simulink model "SoRo_Crt_SMM_20240410"  (R2023a)
settings: Solver=FixedStepAuto  StartTime=0.0  StopTime=50  FixedStep=0.01  RelTol=1e-3
PreLoadFcn:
  | load('traj_pos.mat')
undefined symbols (not defined in the file or in its folder): canChannel
libraries: simulink x18, canmsglib x14, canlib x11, dspfdesign x10, slpidlib x8, auroraNDILibrary x1
(part 1 of 2)
settings Model: Creator=86188  LastModifiedBy=86188
settings DebuggingCC: AlgebraicLoopMsg=none

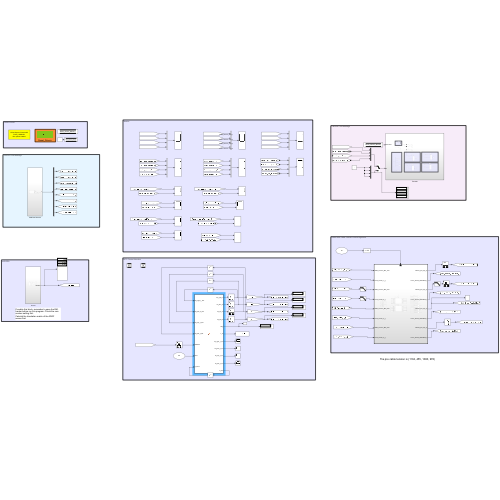
[thumbnail: Simulink's stored preview of the top-level diagram]
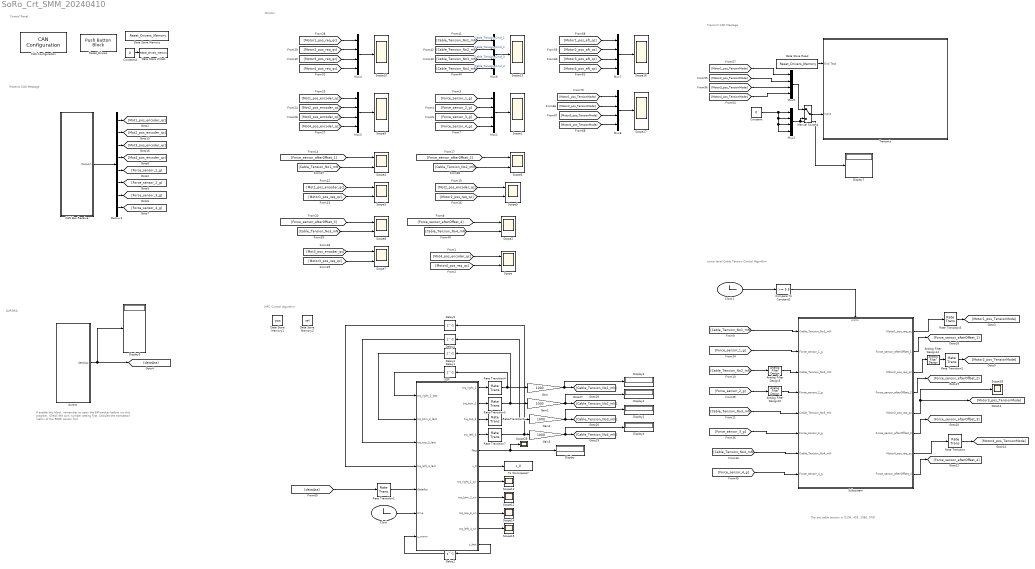
== system SoRo_Crt_SMM_20240410 ==
  note: The pre cable tension is (1104, 455, 1080, 978)
  note: AURORA
  note: If enable this block, remember to open the EM-tracker before run this program. Check the com number setting first.
      | Calculat the translation matrix of the 5DOF sensor first.
  note: Monitor
  note: Control Panel
  note: Lower level Cable Tension Control Algorithm
  note: Receive CAN Message
  note: Transmit CAN Message
  note: MPC Control Algorithm
  Analog Filter Design10 : dspfdesign/Analog Filter Design  method=Butterworth  filttype=Lowpass  N=3  Wlo=20  Whi=80  Rp=2  Rs=40
  Analog Filter Design14 : dspfdesign/Analog Filter Design  method=Butterworth  filttype=Lowpass  N=3  Wlo=20  Whi=80  Rp=2  Rs=40
  Analog Filter Design5 : dspfdesign/Analog Filter Design  method=Butterworth  filttype=Lowpass  N=3  Wlo=20  Whi=80  Rp=2  Rs=40
  Aurora : Subsystem
  CAN Bus Receive : Subsystem
  CAN Configuration : canlib/CAN Configuration  BlockHandle=2496.0005  Device=PEAK-System PCAN-USB (PCAN_USBBUS1)  DeviceMenu=PEAK-System PCAN-USB (PCAN_USBBUS1)  ObjConstructor=canChannel('PEAK-System', 'PCAN_USBBUS1')  BusSpeed=500000  EnableBitParameters=off  AckMode=Normal
  Clock : Clock
  Clock1 : Clock
  Compare To Constant2 : simulink/Logic and Bit Operations/Compare To Constant  relop=>=  const=5.5  OutDataTypeStr=boolean
  Constant : Constant  Value=0
  Constant4 : Constant  Value=0
  Data Store Memory : DataStoreMemory  DataStoreName=Reset_Drivers_Memory  ReadBeforeWriteMsg=warning  WriteAfterWriteMsg=warning  WriteAfterReadMsg=warning  ShowAdditionalParam=off
  Data Store Memory1 : DataStoreMemory  DataStoreName=pos  WriteAfterWriteMsg=warning  InitialValue=pos  ShowAdditionalParam=off  OutDataTypeStr=double
  Data Store Memory2 : DataStoreMemory  DataStoreName=vel  WriteAfterWriteMsg=warning  InitialValue=pos  ShowAdditionalParam=off  OutDataTypeStr=double
  Data Store Read : DataStoreRead  DataStoreName=Reset_Drivers_Memory  DataStoreElements=Reset_Drivers_Memory  IndexOptions=Index vector (dialog)  Indices=1  OutputSizes=1
  Data Store Write1 : DataStoreWrite  DataStoreName=Reset_Drivers_Memory  DataStoreElements=Reset_Drivers_Memory  IndexOptions=Index vector (dialog)  Indices=1  OutputSizes=1
  Delay1 : Delay  DelayLength=1  InitialCondition=0.001
  Delay2 : Delay  DelayLength=1  InitialCondition=|
      | [0.00100000000000000
      | 0.00100000000000000
      | 0.500800000000000
      | 0.00100000000000000
      | 0.00100000000000000
      | 0.00100000000000000
      | 0.500800000000000
      | 0.00100000000000000
      | 0.00100000000000000
      | 0.00100000000000000
      | 0.500800000000000
      | 0.00100000000000000
      | 0.00100000000000000
      | 0.00100000000000000
      | 0.500800000000000
      | 0.00100000000000000
      | 0.00100000000000000
      | 0.00100000000000000
      | 0.500800000000000
      | 0.00100000000000000
      | 0.00100000000000000
      | 0.00100000000000000
      | 0.500800000000000
      | 0.00100000000000000
      | 0.00100000000000000
      | 0.00100000000000000
      | 0.500800000000000
      | 0.00100000000000000
      | 0.00100000000000000
      | 0.00100000000000000
      | 0.500800000000000
      | 0.00100000000000000
      | 0.00100000000000000
      | 0.00100000000000000
      | 0.500800000000000
      | 0.00100000000000000
      | 0.00100000000000000
      | 0.00100000000000000
      | 0.500800000000000
      | 0.00100000000000000
      | -0.136300000000000
      | -0.384000000000000
      | -0.0157000000000000
      | -0.136300000000000
      | -0.384000000000000
      | -0.0157000000000000
      | -0.136300000000000
      | -0.384000000000000
      | -0.0157000000000000
      | -0.136300000000000
      | -0.384000000000000
      | -0.0157000000000000
      | -0.136300000000000
      | -0.384000000000000
      | -0.0157000000000000
      | -0.136300000000000
      | -0.384000000000000
      | -0.0157000000000000
      | -0.136300000000000
      | -0.384000000000000
      | -0.0157000000000000
      | -0.136300000000000
      | -0.384000000000000
      | -0.0157000000000000
      | -0.136300000000000
      | -0.384000000000000
      | -0.0157000000000000
      | -0.136300000000000
      | -0.384000000000000
      | -0.0157000000000000
      | 0
      | 0
      | 0
      | 0
      | 0
      | 0
      | 0
      | 0
      | 0
      | 0]
  Delay3 : Delay  DelayLength=1  InitialCondition=0.001
  Delay4 : Delay  DelayLength=1  InitialCondition=0.5008
  Delay5 : Delay  DelayLength=1  InitialCondition=0.001
  Demux1 : Demux  Outputs=8
  Display{,1..5,7} (7 alike) : Display
  Gain{,1..3} (4 alike) : Gain  Gain=1000
  Manual Switch4 : ManualSwitch
  Mux{1..8} (8 alike) : Mux
  Rate Transition{,2..3,5,7} (5 alike) : RateTransition  OutPortSampleTime=0.01
  Rate Transition1 : RateTransition  OutPortSampleTime=0.05
  Rate Transition4 : RateTransition  InitialCondition=0.001  OutPortSampleTime=0.01
  Rate Transition6 : RateTransition  InitialCondition=0.5008  OutPortSampleTime=0.01
  Reset_Drivers : PushButtonBlock  OffValue=0.000000
  SQP : MATLAB Function  TreatAsAtomicUnit=on
  Scope{,2..8} (8 alike) : Scope  NumInputPorts=2
  Scope{1,9..18,28} (12 alike) : Scope
  Subsystem : Subsystem
  To Workspace7 : ToWorkspace  VariableName=x_0  SaveFormat=Timeseries  SampleTime=-1
  Transmit : Subsystem
  wires:
  CAN Bus Receive/1(Outport) -> Demux1/1
  Constant4/1 -> Data Store Write1/1
  Data Store Read/1 -> Transmit/1(End Test)
  Demux1/1 -> [Mot1_pos_encoder_qc]
  Demux1/2 -> [Mot2_pos_encoder_qc]
  Demux1/3 -> [Mot3_pos_encoder_qc]
  Demux1/4 -> [Mot4_pos_encoder_qc]
  Demux1/5 -> [Force_sensor_1_g]
  Demux1/6 -> [Force_sensor_2_g]
  Demux1/7 -> [Force_sensor_3_g]
  Demux1/8 -> [Force_sensor_4_g]
  Mux2/1 -> Manual Switch4/2, Display7/1
  [Mot4_pos_encoder_qc] -> Scope/1
  [Motor4_pos_req_qc] -> Scope/2
  Constant/1 -> Mux2/3, Mux2/4, Mux2/2, Mux2/1
  [Motor1_pos_req_qc] -> Scope3/2
  [Cable_Tension_No1_mN] -> Scope4/2
  [Force_sensor_afterOffset_1] -> Scope4/1
  [Mot1_pos_encoder_qc] -> Scope3/1
  [Mot2_pos_encoder_qc] -> Scope5/1
  [Motor2_pos_req_qc] -> Scope5/2
  [Mot3_pos_encoder_qc] -> Scope7/1
  [Motor3_pos_req_qc] -> Scope7/2
  [Force_sensor_1_g] -> Mux1/1
  [Force_sensor_2_g] -> Mux1/2
  [Force_sensor_3_g] -> Mux1/3
  [Force_sensor_4_g] -> Mux1/4
  Mux1/1 -> Scope1/1
  Mux3/1 -> Scope9/1
  [Mot4_pos_encoder_qc] -> Mux3/4
  [Mot3_pos_encoder_qc] -> Mux3/3
  [Mot2_pos_encoder_qc] -> Mux3/2
  [Mot1_pos_encoder_qc] -> Mux3/1
  Mux4/1 -> Scope10/1
  [Motor4_pos_req_qc] -> Mux4/4
  [Motor3_pos_req_qc] -> Mux4/3
  [Motor2_pos_req_qc] -> Mux4/2
  [Motor1_pos_req_qc] -> Mux4/1
  Manual Switch4/1 -> Transmit/2(Input)
  Mux5/1 -> Manual Switch4/1
  [Motor2_pos_TensionMode] -> Mux5/2
  [Motor3_pos_TensionMode] -> Mux5/3
  Aurora/1(dataAss) -> Display5/1, [dataAss]
  [Force_sensor_afterOffset_2] -> Scope6/1
  [Cable_Tension_No2_mN] -> Scope6/2
  [Force_sensor_afterOffset_3] -> Scope8/1
  [Cable_Tension_No3_mN] -> Scope8/2
  [Cable_Tension_No4_mN] -> Scope2/2
  [Force_sensor_afterOffset_4] -> Scope2/1
  [Cable_Tension_No1_mN] -> Mux6/1  "Cable_Tension_Cmd_1"
  [Cable_Tension_No2_mN] -> Mux6/2  "Cable_Tension_Cmd_2"
  [Cable_Tension_No3_mN] -> Mux6/3  "Cable_Tension_Cmd_3"
  [Cable_Tension_No4_mN] -> Mux6/4  "Cable_Tension_Cmd_4"
  Mux6/1 -> Scope13/1
  Clock1/1 -> Compare To Constant2/1
  Compare To Constant2/1 -> Subsystem/Enable
  [Cable_Tension_No2_mN] -> Analog Filter Design5/1
  [Force_sensor_2_g] -> Analog Filter Design10/1
  Subsystem/3(Motor2_pos_req_qc) -> Analog Filter Design14/1
  Subsystem/2(Force_sensor_afterOffset_1) -> [Force_sensor_afterOffset_1]
  Subsystem/4(Force_sensor_afterOffset_2) -> [Force_sensor_afterOffset_2]
  Subsystem/6(Force_sensor_afterOffset_3) -> [Force_sensor_afterOffset_3]
  Subsystem/8(Force_sensor_afterOffset_4) -> [Force_sensor_afterOffset_4]
  [Motor1_pos_aft_qc] -> Mux7/1
  [Motor3_pos_aft_qc] -> Mux7/3
  [Motor2_pos_aft_qc] -> Mux7/2
  Mux7/1 -> Scope16/1
  [Motor4_pos_aft_qc] -> Mux7/4
  [Cable_Tension_No1_mN] -> Subsystem/1(Cable_Tension_No1_mN)
  Analog Filter Design5/1 -> Subsystem/3(Cable_Tension_No2_mN)
  [Cable_Tension_No3_mN] -> Subsystem/5(Cable_Tension_No3_mN)
  [Cable_Tension_No4_mN] -> Subsystem/7(Cable_Tension_No4_mN)
  [Force_sensor_1_g] -> Subsystem/2(Force_sensor_1_g)
  Analog Filter Design10/1 -> Subsystem/4(Force_sensor_2_g)
  [Force_sensor_3_g] -> Subsystem/6(Force_sensor_3_g)
  [Force_sensor_4_g] -> Subsystem/8(Force_sensor_4_g)
  [Motor4_pos_TensionMode] -> Mux8/4
  Mux8/1 -> Scope17/1
  [Motor2_pos_TensionMode] -> Mux8/2
  [Motor3_pos_TensionMode] -> Mux8/3
  [Motor1_pos_TensionMode] -> Mux8/1
  Subsystem/1(Motor1_pos_req_qc) -> Rate Transition3/1
  Analog Filter Design14/1 -> Rate Transition2/1
  Subsystem/7(Motor4_pos_req_qc) -> Rate Transition/1
  Rate Transition/1 -> [Motor4_pos_TensionMode]
  Subsystem/5(Motor3_pos_req_qc) -> Scope18/1, [Motor3_pos_TensionMode]
  Rate Transition2/1 -> [Motor2_pos_TensionMode]
  Rate Transition3/1 -> [Motor1_pos_TensionMode]
  [Motor1_pos_TensionMode] -> Mux5/1
  [Motor4_pos_TensionMode] -> Mux5/4
  SQP/1(trq_right_1) -> Rate Transition4/1
  SQP/2(trq_btm_2) -> Rate Transition5/1
  SQP/3(trq_top_3) -> Rate Transition6/1
  SQP/11(z_last) -> Delay2/1
  Clock/1 -> SQP/6(time)
  Delay2/1 -> SQP/7(z_warm)
  SQP/5(flag) -> Display/1, Scope28/1
  SQP/4(trq_left_4) -> Rate Transition7/1
  Rate Transition1/1 -> SQP/5(dataAss)
  Rate Transition4/1 -> Delay1/1, Gain/1
  Rate Transition5/1 -> Delay3/1, Gain1/1
  Rate Transition6/1 -> Delay4/1, Gain2/1
  Rate Transition7/1 -> Delay5/1, Gain3/1
  Gain/1 -> Display3/1, [Cable_Tension_No1_mN]
  Gain1/1 -> [Cable_Tension_No2_mN], Display2/1
  Gain3/1 -> [Cable_Tension_No4_mN], Display4/1
  [dataAss] -> Rate Transition1/1
  SQP/6(x_0) -> To Workspace7/1
  Gain2/1 -> Display1/1, [Cable_Tension_No3_mN]
  Delay1/1 -> SQP/1(trq_right_1_last)
  Delay3/1 -> SQP/2(trq_btm_2_last)
  Delay4/1 -> SQP/3(trq_top_3_last)
  Delay5/1 -> SQP/4(trq_left_4_last)
  SQP/7(trq_right_1_ori) -> Scope11/1
  SQP/8(trq_btm_2_ori) -> Scope12/1
  SQP/9(trq_top_3_ori) -> Scope14/1
  SQP/10(trq_left_4_ori) -> Scope15/1

== system SoRo_Crt_SMM_20240410/Aurora ==
  Aurora NDI Communication : auroraNDILibrary/Aurora NDI Communication  SampleFrequency=20  comNumber=5
  Clock : Clock
  Constant3 : Constant
  Display{1..4} (4 alike) : Display
  Goto5 : Goto  Commented=on  GotoTag=em_tracker_pos  TagVisibility=global
  Subsystem4 : Subsystem
      mask Display: disp('angle of two sensors');
  Subsystem5 : Subsystem  Commented=on
      mask Display: disp('tool1 in tool2');
  Terminator1 : Terminator
  Terminator4 : Terminator
  To Workspace : ToWorkspace  VariableName=DOF5  SaveFormat=Timeseries  SampleTime=-1
  To Workspace1 : ToWorkspace  VariableName=DOF6  SaveFormat=Timeseries  SampleTime=-1
  To Workspace7 : ToWorkspace  VariableName=dataAss  SaveFormat=Timeseries  SampleTime=-1
  t1 : Selector  Commented=on  NumberOfDimensions=2  InputPortWidth=11  IndexOptions=Index vector (dialog),Index vector (dialog)  Indices=[1: 3],4  OutputSizes=1,1
  dataAss : Outport
  wires:
  Aurora NDI Communication/3 -> Terminator1/1
  Aurora NDI Communication/2 -> Display3/1, Subsystem4/2(6DOF), To Workspace1/1
  Constant3/1 -> Aurora NDI Communication/Enable
  Aurora NDI Communication/1 -> Subsystem4/1(5DOF), Display4/1, To Workspace/1
  Aurora NDI Communication/5 -> Display1/1
  Clock/1 -> Aurora NDI Communication/1
  Aurora NDI Communication/4 -> Terminator4/1
  Subsystem5/1(Out1) -> t1/1
  t1/1 -> Goto5/1
  Subsystem4/1(dataAss) -> Display2/1, dataAss/1, To Workspace7/1

== system SoRo_Crt_SMM_20240410/CAN Bus Receive ==
  CAN Receive : canlib/CAN Receive  BlockHandle=2380.0005  Device=PEAK-System PCAN-USB (PCAN_USBBUS1)  DeviceMenu=PEAK-System PCAN-USB (PCAN_USBBUS1)  ObjConstructor=canChannel('PEAK-System', 'PCAN_USBBUS1')  EnableStandardIDsFilter=off  StdIDsCombo=Allow all  StandardIDs=0  EnableExtendedIDsFilter=off  ExtIDsCombo=Allow all  ExtendedIDs=0  SampleTime=0.01  MsgsPerTimestep=all  InternalFilterUpdateStatus=on  BusOutput=on
  Rate Transition : RateTransition  OutPortSampleTime=0.01
  Subsystem : Subsystem
  Outport : Outport
  wires:
  CAN Receive/2 -> Subsystem/1(In2)
  CAN Receive/1 -> Subsystem/Trigger
  Subsystem/1(Outport) -> Rate Transition/1
  Rate Transition/1 -> Outport/1

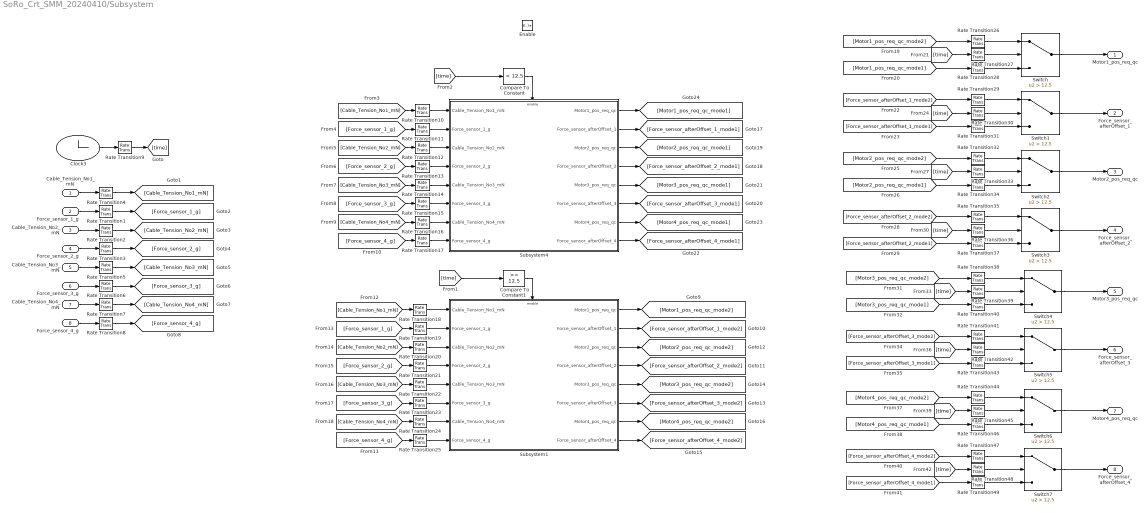
== system SoRo_Crt_SMM_20240410/Subsystem ==
  Cable_Tension_No1_mN : Inport
  Force_sensor_1_g : Inport  Port=2
  Cable_Tension_No2_mN : Inport  Port=3
  Force_sensor_2_g : Inport  Port=4
  Cable_Tension_No3_mN : Inport  Port=5
  Force_sensor_3_g : Inport  Port=6
  Cable_Tension_No4_mN : Inport  Port=7
  Force_sensor_4_g : Inport  Port=8
  Enable : EnablePort
  Clock3 : Clock
  Compare To Constant : simulink/Logic and Bit Operations/Compare To Constant  relop=<  const=12.5  OutDataTypeStr=boolean
  Compare To Constant1 : simulink/Logic and Bit Operations/Compare To Constant  relop=>=  const=12.5  OutDataTypeStr=boolean
  Rate Transition{1..49} (49 alike) : RateTransition  OutPortSampleTime=0.01
  Subsystem1 : Subsystem
  Subsystem4 : Subsystem
  Switch{,1..7} (8 alike) : Switch  Criteria=u2 > Threshold  Threshold=12.5  SaturateOnIntegerOverflow=off  InputSameDT=off
  Motor1_pos_req_qc : Outport
  Force_sensor_afterOffset_1 : Outport  Port=2
  Motor2_pos_req_qc : Outport  Port=3
  Force_sensor_afterOffset_2 : Outport  Port=4
  Motor3_pos_req_qc : Outport  Port=5
  Force_sensor_afterOffset_3 : Outport  Port=6
  Motor4_pos_req_qc : Outport  Port=7
  Force_sensor_afterOffset_4 : Outport  Port=8
  wires:
  Clock3/1 -> Rate Transition9/1
  Compare To Constant/1 -> Subsystem4/Enable
  [time] -> Compare To Constant/1
  Compare To Constant1/1 -> Subsystem1/Enable
  [time] -> Compare To Constant1/1
  [Cable_Tension_No1_mN] -> Rate Transition10/1
  [Force_sensor_1_g] -> Rate Transition11/1
  Cable_Tension_No1_mN/1 -> Rate Transition4/1
  Force_sensor_1_g/1 -> Rate Transition1/1
  Cable_Tension_No2_mN/1 -> Rate Transition2/1
  [Cable_Tension_No2_mN] -> Rate Transition12/1
  [Force_sensor_2_g] -> Rate Transition13/1
  Cable_Tension_No3_mN/1 -> Rate Transition5/1
  Force_sensor_3_g/1 -> Rate Transition6/1
  Cable_Tension_No4_mN/1 -> Rate Transition7/1
  Force_sensor_4_g/1 -> Rate Transition8/1
  Force_sensor_2_g/1 -> Rate Transition3/1
  [Cable_Tension_No3_mN] -> Rate Transition14/1
  [Force_sensor_3_g] -> Rate Transition15/1
  [Cable_Tension_No4_mN] -> Rate Transition16/1
  [Force_sensor_4_g] -> Rate Transition17/1
  [Cable_Tension_No2_mN] -> Rate Transition20/1
  [Force_sensor_2_g] -> Rate Transition21/1
  [Cable_Tension_No3_mN] -> Rate Transition22/1
  [Force_sensor_3_g] -> Rate Transition23/1
  [Cable_Tension_No4_mN] -> Rate Transition24/1
  [Force_sensor_4_g] -> Rate Transition25/1
  [Cable_Tension_No1_mN] -> Rate Transition18/1
  [Force_sensor_1_g] -> Rate Transition19/1
  Switch/1 -> Motor1_pos_req_qc/1
  [Motor1_pos_req_qc_mode2] -> Rate Transition26/1
  [Motor1_pos_req_qc_mode1] -> Rate Transition28/1
  [time] -> Rate Transition27/1
  [Force_sensor_afterOffset_1_mode1] -> Rate Transition31/1
  Switch1/1 -> Force_sensor_afterOffset_1/1
  [time] -> Rate Transition30/1
  [Force_sensor_afterOffset_1_mode2] -> Rate Transition29/1
  [time] -> Rate Transition33/1
  [Motor2_pos_req_qc_mode1] -> Rate Transition34/1
  [Motor2_pos_req_qc_mode2] -> Rate Transition32/1
  Switch2/1 -> Motor2_pos_req_qc/1
  [Force_sensor_afterOffset_2_mode2] -> Rate Transition35/1
  [time] -> Rate Transition36/1
  [Force_sensor_afterOffset_2_mode1] -> Rate Transition37/1
  Switch3/1 -> Force_sensor_afterOffset_2/1
  Switch4/1 -> Motor3_pos_req_qc/1
  [Motor3_pos_req_qc_mode1] -> Rate Transition40/1
  [Force_sensor_afterOffset_3_mode2] -> Rate Transition41/1
  [Motor3_pos_req_qc_mode2] -> Rate Transition38/1
  [time] -> Rate Transition39/1
  [time] -> Rate Transition42/1
  Switch5/1 -> Force_sensor_afterOffset_3/1
  [Force_sensor_afterOffset_3_mode1] -> Rate Transition43/1
  [Motor4_pos_req_qc_mode2] -> Rate Transition44/1
  [time] -> Rate Transition48/1
  [time] -> Rate Transition45/1
  [Force_sensor_afterOffset_4_mode1] -> Rate Transition49/1
  [Force_sensor_afterOffset_4_mode2] -> Rate Transition47/1
  [Motor4_pos_req_qc_mode1] -> Rate Transition46/1
  Switch7/1 -> Force_sensor_afterOffset_4/1
  Switch6/1 -> Motor4_pos_req_qc/1
  Subsystem1/1(Motor1_pos_req_qc) -> [Motor1_pos_req_qc_mode2]
  Subsystem1/2(Force_sensor_afterOffset_1) -> [Force_sensor_afterOffset_1_mode2]
  Subsystem1/3(Motor2_pos_req_qc) -> [Motor2_pos_req_qc_mode2]
  Subsystem1/4(Force_sensor_afterOffset_2) -> [Force_sensor_afterOffset_2_mode2]
  Subsystem1/5(Motor3_pos_req_qc) -> [Motor3_pos_req_qc_mode2]
  Subsystem1/6(Force_sensor_afterOffset_3) -> [Force_sensor_afterOffset_3_mode2]
  Subsystem1/7(Motor4_pos_req_qc) -> [Motor4_pos_req_qc_mode2]
  Subsystem1/8(Force_sensor_afterOffset_4) -> [Force_sensor_afterOffset_4_mode2]
  Subsystem4/1(Motor1_pos_req_qc) -> [Motor1_pos_req_qc_mode1]
  Subsystem4/2(Force_sensor_afterOffset_1) -> [Force_sensor_afterOffset_1_mode1]
  Subsystem4/3(Motor2_pos_req_qc) -> [Motor2_pos_req_qc_mode1]
  Subsystem4/4(Force_sensor_afterOffset_2) -> [Force_sensor_afterOffset_2_mode1]
  Subsystem4/5(Motor3_pos_req_qc) -> [Motor3_pos_req_qc_mode1]
  Subsystem4/6(Force_sensor_afterOffset_3) -> [Force_sensor_afterOffset_3_mode1]
  Subsystem4/7(Motor4_pos_req_qc) -> [Motor4_pos_req_qc_mode1]
  Subsystem4/8(Force_sensor_afterOffset_4) -> [Force_sensor_afterOffset_4_mode1]
  Rate Transition4/1 -> [Cable_Tension_No1_mN]
  Rate Transition1/1 -> [Force_sensor_1_g]
  Rate Transition2/1 -> [Cable_Tension_No2_mN]
  Rate Transition3/1 -> [Force_sensor_2_g]
  Rate Transition5/1 -> [Cable_Tension_No3_mN]
  Rate Transition6/1 -> [Force_sensor_3_g]
  Rate Transition7/1 -> [Cable_Tension_No4_mN]
  Rate Transition8/1 -> [Force_sensor_4_g]
  Rate Transition9/1 -> [time]
  Rate Transition10/1 -> Subsystem4/1(Cable_Tension_No1_mN)
  Rate Transition11/1 -> Subsystem4/2(Force_sensor_1_g)
  Rate Transition12/1 -> Subsystem4/3(Cable_Tension_No2_mN)
  Rate Transition13/1 -> Subsystem4/4(Force_sensor_2_g)
  Rate Transition14/1 -> Subsystem4/5(Cable_Tension_No3_mN)
  Rate Transition15/1 -> Subsystem4/6(Force_sensor_3_g)
  Rate Transition16/1 -> Subsystem4/7(Cable_Tension_No4_mN)
  Rate Transition17/1 -> Subsystem4/8(Force_sensor_4_g)
  Rate Transition18/1 -> Subsystem1/1(Cable_Tension_No1_mN)
  Rate Transition19/1 -> Subsystem1/2(Force_sensor_1_g)
  Rate Transition20/1 -> Subsystem1/3(Cable_Tension_No2_mN)
  Rate Transition21/1 -> Subsystem1/4(Force_sensor_2_g)
  Rate Transition22/1 -> Subsystem1/5(Cable_Tension_No3_mN)
  Rate Transition23/1 -> Subsystem1/6(Force_sensor_3_g)
  Rate Transition24/1 -> Subsystem1/7(Cable_Tension_No4_mN)
  Rate Transition25/1 -> Subsystem1/8(Force_sensor_4_g)
  Rate Transition26/1 -> Switch/1
  Rate Transition27/1 -> Switch/2
  Rate Transition28/1 -> Switch/3
  Rate Transition29/1 -> Switch1/1
  Rate Transition30/1 -> Switch1/2
  Rate Transition31/1 -> Switch1/3
  Rate Transition32/1 -> Switch2/1
  Rate Transition33/1 -> Switch2/2
  Rate Transition34/1 -> Switch2/3
  Rate Transition35/1 -> Switch3/1
  Rate Transition36/1 -> Switch3/2
  Rate Transition37/1 -> Switch3/3
  Rate Transition38/1 -> Switch4/1
  Rate Transition39/1 -> Switch4/2
  Rate Transition40/1 -> Switch4/3
  Rate Transition41/1 -> Switch5/1
  Rate Transition42/1 -> Switch5/2
  Rate Transition43/1 -> Switch5/3
  Rate Transition44/1 -> Switch6/1
  Rate Transition45/1 -> Switch6/2
  Rate Transition46/1 -> Switch6/3
  Rate Transition47/1 -> Switch7/1
  Rate Transition48/1 -> Switch7/2
  Rate Transition49/1 -> Switch7/3

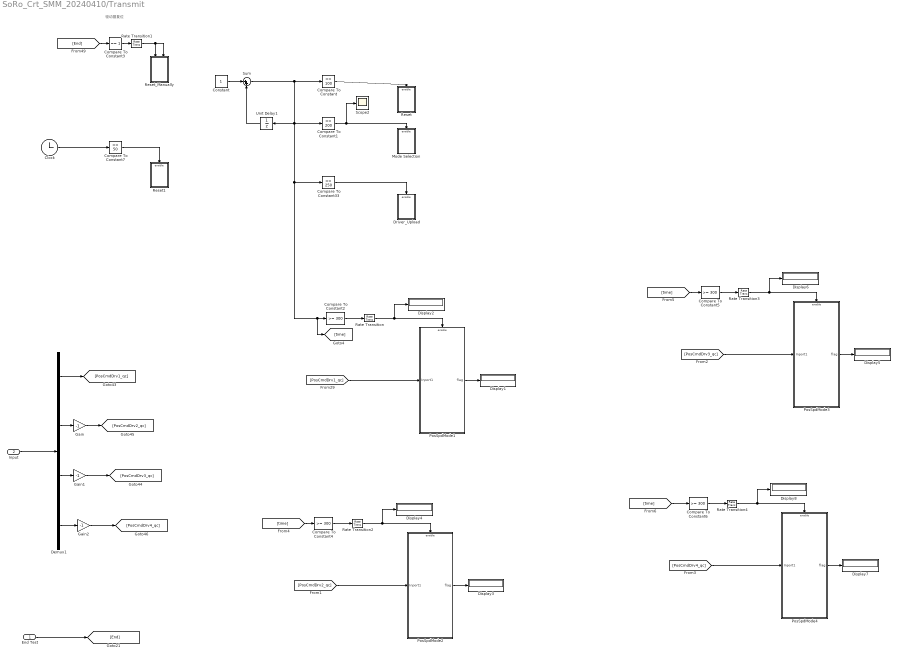
== system SoRo_Crt_SMM_20240410/Transmit ==
  note: 驱动器复位
  End Test : Inport
  Input : Inport  Port=2
  Clock : Clock
  Compare To Constant : simulink/Logic and Bit Operations/Compare To Constant  relop===  const=100  OutDataTypeStr=boolean
  Compare To Constant1 : simulink/Logic and Bit Operations/Compare To Constant  relop===  const=200  OutDataTypeStr=boolean
  Compare To Constant{2,4..6} (4 alike) : simulink/Logic and Bit Operations/Compare To Constant  relop=>=  const=300  OutDataTypeStr=boolean
  Compare To Constant3 : simulink/Logic and Bit Operations/Compare To Constant  relop===  const=1  OutDataTypeStr=boolean
  Compare To Constant33 : simulink/Logic and Bit Operations/Compare To Constant  relop===  const=250  OutDataTypeStr=boolean
  Compare To Constant7 : simulink/Logic and Bit Operations/Compare To Constant  relop===  const=50  OutDataTypeStr=boolean
  Constant : Constant
  Demux1 : Demux
  Display{1..8} (8 alike) : Display
  Driver_Upload : Subsystem
  Gain : Gain  Gain=-1
  Gain1 : Gain  Gain=-1
  Gain2 : Gain  Gain=-1
  Mode Selection : Subsystem  ScheduleAs=Aperiodic partition  PartitionName=TEMP_PRECOMP_PARTITION_NAME_MessageTriggeredSubsystem
  PosSpdMode1 : Subsystem
  PosSpdMode2 : Subsystem
  PosSpdMode3 : Subsystem
  PosSpdMode4 : Subsystem
  Rate Transition{,1..4} (5 alike) : RateTransition  OutPortSampleTime=1
  Reset : Subsystem
  Reset1 : Subsystem
  Reset_Manually : Subsystem
  Scope2 : Scope
  Sum : Sum  Inputs=|++  InputSameDT=on  SaturateOnIntegerOverflow=on  OutDataTypeStr=Inherit: Same as first input
  Unit Delay1 : UnitDelay  SampleTime=-1  HasFrameUpgradeWarning=on
  wires:
  Compare To Constant/1 -> Reset/Enable
  Compare To Constant1/1 -> Scope2/1, Mode Selection/Enable
  Compare To Constant2/1 -> Rate Transition/1
  Constant/1 -> Sum/1
  Unit Delay1/1 -> Sum/2
  Rate Transition/1 -> Display2/1, PosSpdMode1/Enable
  [End] -> Compare To Constant3/1
  [PosCmdDrv1_qc] -> PosSpdMode1/1(Inport1)
  Compare To Constant3/1 -> Rate Transition1/1
  Rate Transition1/1 -> Reset_Manually/Trigger, Reset_Manually/Enable
  Demux1/1 -> [PosCmdDrv1_qc]
  Demux1/3 -> Gain1/1
  Demux1/4 -> Gain2/1
  Input/1 -> Demux1/1
  Demux1/2 -> Gain/1
  End Test/1 -> [End]
  PosSpdMode1/1(flag) -> Display1/1
  PosSpdMode2/1(flag) -> Display3/1
  [PosCmdDrv2_qc] -> PosSpdMode2/1(Inport1)
  Rate Transition2/1 -> Display4/1, PosSpdMode2/Enable
  Compare To Constant4/1 -> Rate Transition2/1
  PosSpdMode3/1(flag) -> Display5/1
  [PosCmdDrv3_qc] -> PosSpdMode3/1(Inport1)
  Rate Transition3/1 -> Display6/1, PosSpdMode3/Enable
  Compare To Constant5/1 -> Rate Transition3/1
  PosSpdMode4/1(flag) -> Display7/1
  [PosCmdDrv4_qc] -> PosSpdMode4/1(Inport1)
  Rate Transition4/1 -> Display8/1, PosSpdMode4/Enable
  Compare To Constant6/1 -> Rate Transition4/1
  [time] -> Compare To Constant4/1
  [time] -> Compare To Constant5/1
  [time] -> Compare To Constant6/1
  Compare To Constant33/1 -> Driver_Upload/Enable
  Sum/1 -> [time], Compare To Constant2/1, Compare To Constant33/1, Compare To Constant1/1, Unit Delay1/1, Compare To Constant/1
  Gain/1 -> [PosCmdDrv2_qc]
  Gain1/1 -> [PosCmdDrv3_qc]
  Gain2/1 -> [PosCmdDrv4_qc]
  Compare To Constant7/1 -> Reset1/Enable
  Clock/1 -> Compare To Constant7/1

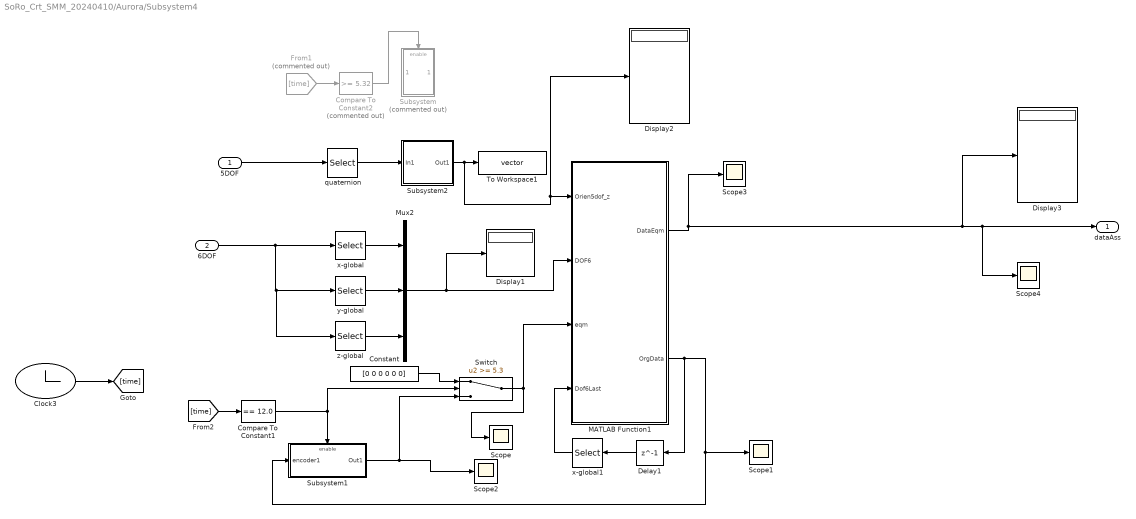
== system SoRo_Crt_SMM_20240410/Aurora/Subsystem4 ==
  5DOF : Inport
  6DOF : Inport  Port=2
  Clock3 : Clock
  Compare To Constant1 : simulink/Logic and Bit Operations/Compare To Constant  relop===  const=12.0  OutDataTypeStr=boolean
  Compare To Constant2 : simulink/Logic and Bit Operations/Compare To Constant  Commented=on  relop=>=  const=5.32  OutDataTypeStr=boolean
  Constant : Constant  Value=|
      | [0
      | 0
      | 0
      | 0
      | 0
      | 0]
  Delay1 : Delay  DelayLength=1  InitialCondition=[0; 0; 0; 0; 0; 0]
  Display1 : Display
  Display2 : Display
  Display3 : Display
  From1 : From  Commented=on  GotoTag=time
  MATLAB Function1 : MATLAB Function  TreatAsAtomicUnit=on
  Mux2 : Mux  Inputs=3
  Scope{,1..4} (5 alike) : Scope
  Subsystem : Subsystem  Commented=on
  Subsystem1 : Subsystem
  Subsystem2 : Subsystem
      mask Display: disp('z vector');
  Switch : Switch  Threshold=5.3  SaturateOnIntegerOverflow=off  InputSameDT=off
  To Workspace1 : ToWorkspace  VariableName=vector  SaveFormat=Timeseries  SampleTime=-1
  quaternion : Selector  InputPortWidth=7  IndexOptions=Index vector (dialog)  Indices=[1: 4]  OutputSizes=1
  x-global : Selector  InputPortWidth=7  IndexOptions=Index vector (dialog)  Indices=[5]  OutputSizes=1
  x-global1 : Selector  InputPortWidth=6  IndexOptions=Index vector (dialog)  Indices=[4:6]  OutputSizes=1
  y-global : Selector  InputPortWidth=7  IndexOptions=Index vector (dialog)  Indices=[6]  OutputSizes=1
  z-global : Selector  InputPortWidth=7  IndexOptions=Index vector (dialog)  Indices=[7]  OutputSizes=1
  dataAss : Outport
  wires:
  Subsystem2/1(Out1) -> Display2/1, MATLAB Function1/1(Orien5dof_z), To Workspace1/1
  quaternion/1 -> Subsystem2/1(In1)
  x-global/1 -> Mux2/1
  y-global/1 -> Mux2/2
  z-global/1 -> Mux2/3
  Switch/1 -> Scope/1, MATLAB Function1/3(eqm)
  6DOF/1 -> z-global/1, y-global/1, x-global/1
  5DOF/1 -> quaternion/1
  Compare To Constant1/1 -> Switch/2, Subsystem1/Enable
  [time] -> Compare To Constant1/1
  Mux2/1 -> Display1/1, MATLAB Function1/2(DOF6)
  MATLAB Function1/2(OrgData) -> Delay1/1, Subsystem1/1(encoder1), Scope1/1
  Subsystem1/1(Out1) -> Switch/3, Scope2/1
  Clock3/1 -> [time]
  Constant/1 -> Switch/1
  From1/1 -> Compare To Constant2/1
  Compare To Constant2/1 -> Subsystem/Enable
  MATLAB Function1/1(DataEqm) -> Display3/1, Scope4/1, dataAss/1, Scope3/1
  Delay1/1 -> x-global1/1
  x-global1/1 -> MATLAB Function1/4(Dof6Last)

== system SoRo_Crt_SMM_20240410/Aurora/Subsystem5 ==
  In1 : Inport
  In2 : Inport  Port=2
  Constant : Constant  Value=[0 0 0 1]  VectorParams1D=off
  Constant1 : Constant  Value=[0 0 0 1]  VectorParams1D=off
  Divide : Product  Inputs=*/  Multiplication=Matrix(*)
  Matrix Concatenate : Concatenate  Mode=Multidimensional array  ConcatenateDimension=2
  Matrix Concatenate1 : Concatenate  Mode=Multidimensional array
  Matrix Concatenate2 : Concatenate  Mode=Multidimensional array  ConcatenateDimension=2
  Matrix Concatenate3 : Concatenate  Mode=Multidimensional array
  Subsystem2 : Subsystem
      mask Display: disp('q2rot');
  Subsystem3 : Subsystem
      mask Display: disp('q2rot');
  q1 : Selector  InputPortWidth=11  IndexOptions=Index vector (dialog)  Indices=[4: 7]  OutputSizes=1
  q2 : Selector  InputPortWidth=11  IndexOptions=Index vector (dialog)  Indices=[4: 7]  OutputSizes=1
  t1 : Selector  InputPortWidth=11  IndexOptions=Index vector (dialog)  Indices=[8: 10]  OutputSizes=1
  t2 : Selector  InputPortWidth=11  IndexOptions=Index vector (dialog)  Indices=[8: 10]  OutputSizes=1
  Out1 : Outport
  wires:
  In2/1 -> t2/1, q2/1
  q2/1 -> Subsystem3/1(In1)
  q1/1 -> Subsystem2/1(In1)
  In1/1 -> t1/1, q1/1
  Subsystem2/1(Out1) -> Matrix Concatenate/1
  t1/1 -> Matrix Concatenate/2
  Matrix Concatenate/1 -> Matrix Concatenate1/1
  Constant/1 -> Matrix Concatenate1/2
  Constant1/1 -> Matrix Concatenate3/2
  Matrix Concatenate2/1 -> Matrix Concatenate3/1
  t2/1 -> Matrix Concatenate2/2
  Subsystem3/1(Out1) -> Matrix Concatenate2/1
  Matrix Concatenate1/1 -> Divide/1
  Matrix Concatenate3/1 -> Divide/2
  Divide/1 -> Out1/1

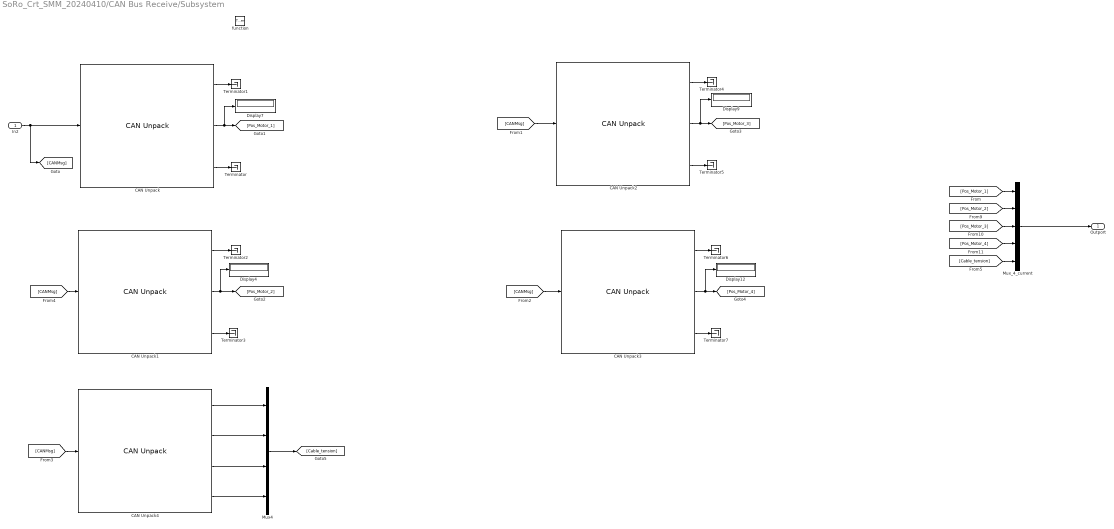
== system SoRo_Crt_SMM_20240410/CAN Bus Receive/Subsystem ==
  In2 : Inport
  function : TriggerPort  TriggerType=function-call  VariantControl=Variant
  CAN Unpack : canmsglib/CAN Unpack  CANdbFile=E:\Research\SRIL\9th\Mnp_Control_Sim\RoboModule0611.dbc  MsgList=Feedback_curvelpos_Dv1  MsgName=Feedback_curvelpos_Dv1  MsgIDType=Standard (11-bit identifier)  MsgIdentifier=27  MsgLength=8  SignalInfo={'real_current','8','16','BE','signed','Standard','0','1','0','-Inf','Inf';'real_position','56','32','BE','signed','Standard','0','1','0','-Inf','Inf';'real_velocity','24','16','BE','signed','Standard','0','1','0','-Inf','Inf'}  IDPort=off  TimestampPort=off  ErrorPort=off  RemotePort=off  LengthPort=off  StatusPort=off  ApplyMinMax=off
      settings: DataFormat=CANdb specified signals
  CAN Unpack1 : canmsglib/CAN Unpack  CANdbFile=E:\Research\SRIL\9th\Mnp_Control_Sim\RoboModule0611.dbc  MsgList=Feedback_curvelpos_Dv2  MsgName=Feedback_curvelpos_Dv2  MsgIDType=Standard (11-bit identifier)  MsgIdentifier=43  MsgLength=8  SignalInfo={'real_current','8','16','BE','signed','Standard','0','1','0','-Inf','Inf';'real_position','56','32','BE','signed','Standard','0','1','0','-Inf','Inf';'real_velocity','24','16','BE','signed','Standard','0','1','0','-Inf','Inf'}  IDPort=off  TimestampPort=off  ErrorPort=off  RemotePort=off  LengthPort=off  StatusPort=off  ApplyMinMax=off
      settings: DataFormat=CANdb specified signals
  CAN Unpack2 : canmsglib/CAN Unpack  CANdbFile=E:\Research\SRIL\9th\Mnp_Control_Sim\RoboModule0611.dbc  MsgList=Feedback_curvelpos_Dv3  MsgName=Feedback_curvelpos_Dv3  MsgIDType=Standard (11-bit identifier)  MsgIdentifier=59  MsgLength=8  SignalInfo={'real_current','8','16','BE','signed','Standard','0','1','0','-Inf','Inf';'real_position','56','32','BE','signed','Standard','0','1','0','-Inf','Inf';'real_velocity','24','16','BE','signed','Standard','0','1','0','-Inf','Inf'}  IDPort=off  TimestampPort=off  ErrorPort=off  RemotePort=off  LengthPort=off  StatusPort=off  ApplyMinMax=off
      settings: DataFormat=CANdb specified signals
  CAN Unpack3 : canmsglib/CAN Unpack  CANdbFile=E:\Research\SRIL\9th\Mnp_Control_Sim\RoboModule0611.dbc  MsgList=Feedback_curvelpos_Dr4  MsgName=Feedback_curvelpos_Dr4  MsgIDType=Standard (11-bit identifier)  MsgIdentifier=75  MsgLength=8  SignalInfo={'real_current','8','16','BE','signed','Standard','0','1','0','-Inf','Inf';'real_position','56','32','BE','signed','Standard','0','1','0','-Inf','Inf';'real_velocity','24','16','BE','signed','Standard','0','1','0','-Inf','Inf'}  IDPort=off  TimestampPort=off  ErrorPort=off  RemotePort=off  LengthPort=off  StatusPort=off  ApplyMinMax=off
      settings: DataFormat=CANdb specified signals
  CAN Unpack4 : canmsglib/CAN Unpack  CANdbFile=E:\Research\SRIL\9th\Mnp_Control_Sim\RoboModule0611.dbc  MsgList=Cable_tension  MsgName=Cable_tension  MsgIDType=Extended (29-bit identifier)  MsgIdentifier=529024  MsgLength=8  SignalInfo={ 'Force_sensor_1', '8', '16', 'BE', 'signed', 'Standard', '0', '1', '0', '-Inf', 'Inf'; 'Force_sensor_2', '24', '16', 'BE', 'signed', 'Standard', '0', '1', '0', '-Inf', 'Inf'; 'Force_sensor_3', '40', '16', 'BE', 'signed', 'Standard', '0', '1', '0', '-Inf', 'Inf'; 'Force_sensor_4', '56', '16', 'BE', 'signed', 'Standard', '0', '1', '0', '-Inf', 'Inf' }  IDPort=off  TimestampPort=off  ErrorPort=off  RemotePort=off  LengthPort=off  StatusPort=off  ApplyMinMax=off
  Display{4,7,9,12} (4 alike) : Display
      settings: Format=hex (Stored Integer)
  Mux4 : Mux
  Mux_4_current : Mux  Inputs=5
  Terminator{,1..7} (8 alike) : Terminator
  Outport : Outport
  wires:
  CAN Unpack3/3 -> Terminator7/1
  CAN Unpack2/2 -> [Pos_Motor_3], Display9/1
  [CANMsg] -> CAN Unpack2/1
  CAN Unpack2/1 -> Terminator4/1
  In2/1 -> CAN Unpack/1, [CANMsg]
  CAN Unpack3/2 -> [Pos_Motor_4], Display12/1
  [CANMsg] -> CAN Unpack3/1
  CAN Unpack2/3 -> Terminator5/1
  CAN Unpack1/1 -> Terminator2/1
  CAN Unpack/3 -> Terminator/1
  CAN Unpack/1 -> Terminator1/1
  CAN Unpack/2 -> Display7/1, [Pos_Motor_1]
  CAN Unpack1/2 -> [Pos_Motor_2], Display4/1
  CAN Unpack1/3 -> Terminator3/1
  [Pos_Motor_1] -> Mux_4_current/1
  [Pos_Motor_4] -> Mux_4_current/4
  [Pos_Motor_3] -> Mux_4_current/3
  [Pos_Motor_2] -> Mux_4_current/2
  [CANMsg] -> CAN Unpack4/1
  [CANMsg] -> CAN Unpack1/1
  CAN Unpack4/1 -> Mux4/1
  CAN Unpack4/2 -> Mux4/2
  CAN Unpack4/3 -> Mux4/3
  CAN Unpack4/4 -> Mux4/4
  Mux4/1 -> [Cable_tension]
  [Cable_tension] -> Mux_4_current/5
  CAN Unpack3/1 -> Terminator6/1
  Mux_4_current/1 -> Outport/1

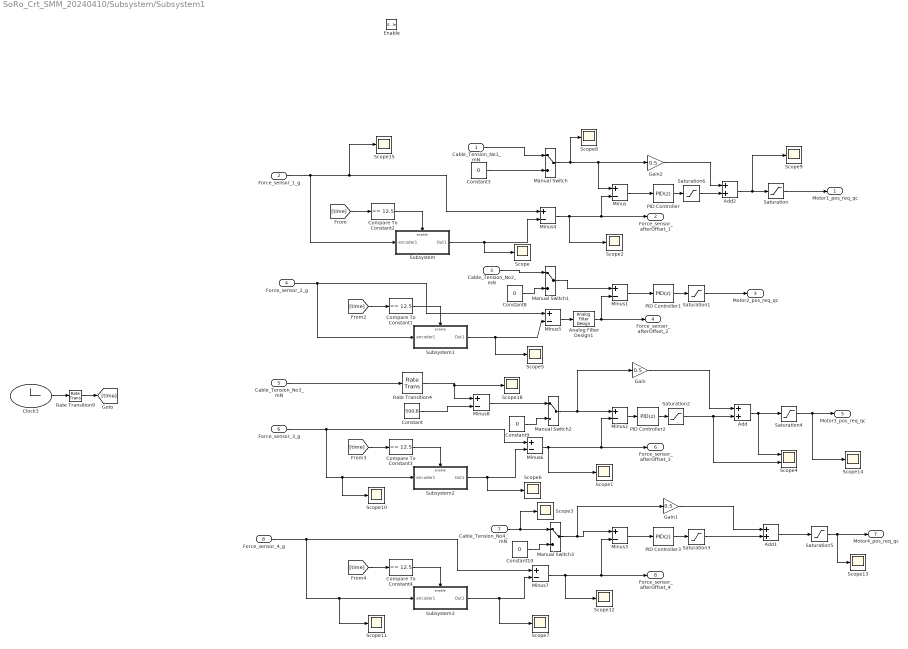
== system SoRo_Crt_SMM_20240410/Subsystem/Subsystem1 ==
  Cable_Tension_No1_mN : Inport
  Force_sensor_1_g : Inport  Port=2
  Cable_Tension_No2_mN : Inport  Port=3
  Force_sensor_2_g : Inport  Port=4
  Cable_Tension_No3_mN : Inport  Port=5
  Force_sensor_3_g : Inport  Port=6
  Cable_Tension_No4_mN : Inport  Port=7
  Force_sensor_4_g : Inport  Port=8
  Enable : EnablePort
  Add : Sum
  Add1 : Sum
  Add2 : Sum
  Analog Filter Design1 : dspfdesign/Analog Filter Design  method=Chebyshev I  filttype=Lowpass  N=3  Wlo=1.5  Whi=80  Rp=2  Rs=40
  Clock3 : Clock
  Compare To Constant{1..4} (4 alike) : simulink/Logic and Bit Operations/Compare To Constant  relop===  const=12.5  OutDataTypeStr=boolean
  Constant : Constant  Value=500.8
  Constant{3,8..10} (4 alike) : Constant  Value=0  SampleTime=0.01
  Gain : Gain  Gain=0.5
  Gain1 : Gain  Gain=0.5
  Gain2 : Gain  Gain=0.5
  Manual Switch{,1..3} (4 alike) : ManualSwitch
  Minus{,1..8} (9 alike) : Sum  Inputs=+-
  PID Controller : slpidlib/PID Controller  Controller=PID  Form=Parallel  TimeDomain=Discrete-time  UseExternalTs=off  SampleTime=-1  IntegratorMethod=Forward Euler  FilterMethod=Forward Euler  ControllerParametersSource=internal  P=0.2  I=0  UseKiTs=off  D=0  N=100  UseFilter=on  TunerSelectOption=Transfer Function Based (PID Tuner App)  InitialConditionSource=internal  InitialConditionForIntegrator=0  InitialConditionForFilter=0  DifferentiatorICPrevScaledInput=0  ExternalReset=none  TrackingMode=off  Kt=1  LimitOutput=off  SatLimitsSource=internal  UpperSaturationLimit=inf  LowerSaturationLimit=-inf  LinearizeAsGain=on  AntiWindupMode=none  Kb=1  LimitIntegrator=off  UpperIntegratorSaturationLimit=inf  LowerIntegratorSaturationLimit=-inf  POutMin=[]  POutMax=[]  IOutMin=[]  IOutMax=[]  DOutMin=[]  DOutMax=[]  NOutMin=[]  NOutMax=[]  SumOutMin=[]  SumOutMax=[]  SaturationOutMin=[]  SaturationOutMax=[]  PParamMin=[]  PParamMax=[]  IParamMin=[]  IParamMax=[]  DParamMin=[]  DParamMax=[]  NParamMin=[]  NParamMax=[]  KbParamMin=[]  KbParamMax=[]  KtParamMin=[]  KtParamMax=[]  KbOutMin=[]  KbOutMax=[]  KtOutMin=[]  KtOutMax=[]  IntegratorOutMin=[]  IntegratorOutMax=[]  FilterOutMin=[]  FilterOutMax=[]  SumI1OutMin=[]  SumI1OutMax=[]  SumI2OutMin=[]  SumI2OutMax=[]  SumI3OutMin=[]  SumI3OutMax=[]  SumI4OutMin=[]  SumI4OutMax=[]  SumDOutMin=[]  SumDOutMax=[]  DifferentiatorOutMin=[]  DifferentiatorOutMax=[]  FilterDiffOutCoefMin=[]  FilterDiffOutCoefMax=[]  ReciprocalOutMin=[]  ReciprocalOutMax=[]  SumDenOutMin=[]  SumDenOutMax=[]  SumNumOutMin=[]  SumNumOutMax=[]  DivideOutMin=[]  DivideOutMax=[]  UdiffTsProdOutMin=[]  UdiffTsProdOutMax=[]  NTsProdOutMin=[]  NTsProdOutMax=[]  UintegralTsProdOutMin=[]  UintegralTsProdOutMax=[]  UngainTsProdOutMin=[]  UngainTsProdOutMax=[]  ClampingZeroOutDataTypeStr=Inherit: Inherit via back propagation  ClampingZeroOutMin=[]  ClampingZeroOutMax=[]  FilterDenConstantOutDataTypeStr=Inherit: Inherit via back propagation  FilterDenConstantOutMin=[]  FilterDenConstantOutMax=[]  PCopyOutDataTypeStr=Inherit: Inherit via back propagation  PCopyOutMin=[]  PCopyOutMax=[]  NCopyOutDataTypeStr=Inherit: Inherit via back propagation  NCopyOutMin=[]  NCopyOutMax=[]  IntegratorContinuousStateAttributes=''  IntegratorStateMustResolveToSignalObject=off  IntegratorRTWStateStorageClass=Auto  FilterContinuousStateAttributes=''  FilterStateMustResolveToSignalObject=off  FilterRTWStateStorageClass=Auto  ParallelPVariant=InternalParameters  IdealPVariant=Disabled  IVariant=InternalParameters  DVariant=InternalParameters  IntegratorVariant=Discrete  SatVariant=Disabled  AWVariant=Passthrough  PCopyVariant=Disabled  TRVariant=Disabled  FdbkBlocksVariant=Forward  IdealPFdbkVariant=Disabled  SatFdbkVariant=Disabled  DerivativeFilterVariant=ForwardEulerFilter  NVariant=InternalParameters  NCopyVariant=Disabled  FilterICVariant=InternalICsFilter  IntegratorICVariant=InternalICs  ExternalResetVariant=Disabled  TRSumVariant=Passthrough  SumFdbkVariant=Disabled  SumVariant=Sum_PID  TsampFilterVariant=InternalTs  TsampNgainVariant=Passthrough  TsampIntegralVariant=Disabled_SignalSpec  ExternalSaturationOutDataTypeStr=Inherit: Same as second input
  PID Controller1 : slpidlib/PID Controller  Controller=PID  Form=Parallel  TimeDomain=Discrete-time  UseExternalTs=off  SampleTime=-1  IntegratorMethod=Forward Euler  FilterMethod=Forward Euler  ControllerParametersSource=internal  P=0.4  I=0  UseKiTs=off  D=0  N=100  UseFilter=on  TunerSelectOption=Transfer Function Based (PID Tuner App)  InitialConditionSource=internal  InitialConditionForIntegrator=0  InitialConditionForFilter=0  DifferentiatorICPrevScaledInput=0  ExternalReset=none  TrackingMode=off  Kt=1  LimitOutput=off  SatLimitsSource=internal  UpperSaturationLimit=inf  LowerSaturationLimit=-inf  LinearizeAsGain=on  AntiWindupMode=none  Kb=1  LimitIntegrator=off  UpperIntegratorSaturationLimit=inf  LowerIntegratorSaturationLimit=-inf  POutMin=[]  POutMax=[]  IOutMin=[]  IOutMax=[]  DOutMin=[]  DOutMax=[]  NOutMin=[]  NOutMax=[]  SumOutMin=[]  SumOutMax=[]  SaturationOutMin=[]  SaturationOutMax=[]  PParamMin=[]  PParamMax=[]  IParamMin=[]  IParamMax=[]  DParamMin=[]  DParamMax=[]  NParamMin=[]  NParamMax=[]  KbParamMin=[]  KbParamMax=[]  KtParamMin=[]  KtParamMax=[]  KbOutMin=[]  KbOutMax=[]  KtOutMin=[]  KtOutMax=[]  IntegratorOutMin=[]  IntegratorOutMax=[]  FilterOutMin=[]  FilterOutMax=[]  SumI1OutMin=[]  SumI1OutMax=[]  SumI2OutMin=[]  SumI2OutMax=[]  SumI3OutMin=[]  SumI3OutMax=[]  SumI4OutMin=[]  SumI4OutMax=[]  SumDOutMin=[]  SumDOutMax=[]  DifferentiatorOutMin=[]  DifferentiatorOutMax=[]  FilterDiffOutCoefMin=[]  FilterDiffOutCoefMax=[]  ReciprocalOutMin=[]  ReciprocalOutMax=[]  SumDenOutMin=[]  SumDenOutMax=[]  SumNumOutMin=[]  SumNumOutMax=[]  DivideOutMin=[]  DivideOutMax=[]  UdiffTsProdOutMin=[]  UdiffTsProdOutMax=[]  NTsProdOutMin=[]  NTsProdOutMax=[]  UintegralTsProdOutMin=[]  UintegralTsProdOutMax=[]  UngainTsProdOutMin=[]  UngainTsProdOutMax=[]  ClampingZeroOutDataTypeStr=Inherit: Inherit via back propagation  ClampingZeroOutMin=[]  ClampingZeroOutMax=[]  FilterDenConstantOutDataTypeStr=Inherit: Inherit via back propagation  FilterDenConstantOutMin=[]  FilterDenConstantOutMax=[]  PCopyOutDataTypeStr=Inherit: Inherit via back propagation  PCopyOutMin=[]  PCopyOutMax=[]  NCopyOutDataTypeStr=Inherit: Inherit via back propagation  NCopyOutMin=[]  NCopyOutMax=[]  IntegratorContinuousStateAttributes=''  IntegratorStateMustResolveToSignalObject=off  IntegratorRTWStateStorageClass=Auto  FilterContinuousStateAttributes=''  FilterStateMustResolveToSignalObject=off  FilterRTWStateStorageClass=Auto  ParallelPVariant=InternalParameters  IdealPVariant=Disabled  IVariant=InternalParameters  DVariant=InternalParameters  IntegratorVariant=Discrete  SatVariant=Disabled  AWVariant=Passthrough  PCopyVariant=Disabled  TRVariant=Disabled  FdbkBlocksVariant=Forward  IdealPFdbkVariant=Disabled  SatFdbkVariant=Disabled  DerivativeFilterVariant=ForwardEulerFilter  NVariant=InternalParameters  NCopyVariant=Disabled  FilterICVariant=InternalICsFilter  IntegratorICVariant=InternalICs  ExternalResetVariant=Disabled  TRSumVariant=Passthrough  SumFdbkVariant=Disabled  SumVariant=Sum_PID  TsampFilterVariant=InternalTs  TsampNgainVariant=Passthrough  TsampIntegralVariant=Disabled_SignalSpec  ExternalSaturationOutDataTypeStr=Inherit: Same as second input
  PID Controller2 : slpidlib/PID Controller  Controller=PID  Form=Parallel  TimeDomain=Discrete-time  UseExternalTs=off  SampleTime=-1  IntegratorMethod=Forward Euler  FilterMethod=Forward Euler  ControllerParametersSource=internal  P=0.2  I=0  UseKiTs=off  D=0  N=100  UseFilter=on  TunerSelectOption=Transfer Function Based (PID Tuner App)  InitialConditionSource=internal  InitialConditionForIntegrator=0  InitialConditionForFilter=0  DifferentiatorICPrevScaledInput=0  ExternalReset=none  TrackingMode=off  Kt=1  LimitOutput=off  SatLimitsSource=internal  UpperSaturationLimit=inf  LowerSaturationLimit=-inf  LinearizeAsGain=on  AntiWindupMode=none  Kb=1  LimitIntegrator=off  UpperIntegratorSaturationLimit=inf  LowerIntegratorSaturationLimit=-inf  POutMin=[]  POutMax=[]  IOutMin=[]  IOutMax=[]  DOutMin=[]  DOutMax=[]  NOutMin=[]  NOutMax=[]  SumOutMin=[]  SumOutMax=[]  SaturationOutMin=[]  SaturationOutMax=[]  PParamMin=[]  PParamMax=[]  IParamMin=[]  IParamMax=[]  DParamMin=[]  DParamMax=[]  NParamMin=[]  NParamMax=[]  KbParamMin=[]  KbParamMax=[]  KtParamMin=[]  KtParamMax=[]  KbOutMin=[]  KbOutMax=[]  KtOutMin=[]  KtOutMax=[]  IntegratorOutMin=[]  IntegratorOutMax=[]  FilterOutMin=[]  FilterOutMax=[]  SumI1OutMin=[]  SumI1OutMax=[]  SumI2OutMin=[]  SumI2OutMax=[]  SumI3OutMin=[]  SumI3OutMax=[]  SumI4OutMin=[]  SumI4OutMax=[]  SumDOutMin=[]  SumDOutMax=[]  DifferentiatorOutMin=[]  DifferentiatorOutMax=[]  FilterDiffOutCoefMin=[]  FilterDiffOutCoefMax=[]  ReciprocalOutMin=[]  ReciprocalOutMax=[]  SumDenOutMin=[]  SumDenOutMax=[]  SumNumOutMin=[]  SumNumOutMax=[]  DivideOutMin=[]  DivideOutMax=[]  UdiffTsProdOutMin=[]  UdiffTsProdOutMax=[]  NTsProdOutMin=[]  NTsProdOutMax=[]  UintegralTsProdOutMin=[]  UintegralTsProdOutMax=[]  UngainTsProdOutMin=[]  UngainTsProdOutMax=[]  ClampingZeroOutDataTypeStr=Inherit: Inherit via back propagation  ClampingZeroOutMin=[]  ClampingZeroOutMax=[]  FilterDenConstantOutDataTypeStr=Inherit: Inherit via back propagation  FilterDenConstantOutMin=[]  FilterDenConstantOutMax=[]  PCopyOutDataTypeStr=Inherit: Inherit via back propagation  PCopyOutMin=[]  PCopyOutMax=[]  NCopyOutDataTypeStr=Inherit: Inherit via back propagation  NCopyOutMin=[]  NCopyOutMax=[]  IntegratorContinuousStateAttributes=''  IntegratorStateMustResolveToSignalObject=off  IntegratorRTWStateStorageClass=Auto  FilterContinuousStateAttributes=''  FilterStateMustResolveToSignalObject=off  FilterRTWStateStorageClass=Auto  ParallelPVariant=InternalParameters  IdealPVariant=Disabled  IVariant=InternalParameters  DVariant=InternalParameters  IntegratorVariant=Discrete  SatVariant=Disabled  AWVariant=Passthrough  PCopyVariant=Disabled  TRVariant=Disabled  FdbkBlocksVariant=Forward  IdealPFdbkVariant=Disabled  SatFdbkVariant=Disabled  DerivativeFilterVariant=ForwardEulerFilter  NVariant=InternalParameters  NCopyVariant=Disabled  FilterICVariant=InternalICsFilter  IntegratorICVariant=InternalICs  ExternalResetVariant=Disabled  TRSumVariant=Passthrough  SumFdbkVariant=Disabled  SumVariant=Sum_PID  TsampFilterVariant=InternalTs  TsampNgainVariant=Passthrough  TsampIntegralVariant=Disabled_SignalSpec  ExternalSaturationOutDataTypeStr=Inherit: Same as second input
  PID Controller3 : slpidlib/PID Controller  Controller=PID  Form=Parallel  TimeDomain=Discrete-time  UseExternalTs=off  SampleTime=-1  IntegratorMethod=Forward Euler  FilterMethod=Forward Euler  ControllerParametersSource=internal  P=0.3  I=0  UseKiTs=off  D=0  N=100  UseFilter=on  TunerSelectOption=Transfer Function Based (PID Tuner App)  InitialConditionSource=internal  InitialConditionForIntegrator=0  InitialConditionForFilter=0  DifferentiatorICPrevScaledInput=0  ExternalReset=none  TrackingMode=off  Kt=1  LimitOutput=off  SatLimitsSource=internal  UpperSaturationLimit=inf  LowerSaturationLimit=-inf  LinearizeAsGain=on  AntiWindupMode=none  Kb=1  LimitIntegrator=off  UpperIntegratorSaturationLimit=inf  LowerIntegratorSaturationLimit=-inf  POutMin=[]  POutMax=[]  IOutMin=[]  IOutMax=[]  DOutMin=[]  DOutMax=[]  NOutMin=[]  NOutMax=[]  SumOutMin=[]  SumOutMax=[]  SaturationOutMin=[]  SaturationOutMax=[]  PParamMin=[]  PParamMax=[]  IParamMin=[]  IParamMax=[]  DParamMin=[]  DParamMax=[]  NParamMin=[]  NParamMax=[]  KbParamMin=[]  KbParamMax=[]  KtParamMin=[]  KtParamMax=[]  KbOutMin=[]  KbOutMax=[]  KtOutMin=[]  KtOutMax=[]  IntegratorOutMin=[]  IntegratorOutMax=[]  FilterOutMin=[]  FilterOutMax=[]  SumI1OutMin=[]  SumI1OutMax=[]  SumI2OutMin=[]  SumI2OutMax=[]  SumI3OutMin=[]  SumI3OutMax=[]  SumI4OutMin=[]  SumI4OutMax=[]  SumDOutMin=[]  SumDOutMax=[]  DifferentiatorOutMin=[]  DifferentiatorOutMax=[]  FilterDiffOutCoefMin=[]  FilterDiffOutCoefMax=[]  ReciprocalOutMin=[]  ReciprocalOutMax=[]  SumDenOutMin=[]  SumDenOutMax=[]  SumNumOutMin=[]  SumNumOutMax=[]  DivideOutMin=[]  DivideOutMax=[]  UdiffTsProdOutMin=[]  UdiffTsProdOutMax=[]  NTsProdOutMin=[]  NTsProdOutMax=[]  UintegralTsProdOutMin=[]  UintegralTsProdOutMax=[]  UngainTsProdOutMin=[]  UngainTsProdOutMax=[]  ClampingZeroOutDataTypeStr=Inherit: Inherit via back propagation  ClampingZeroOutMin=[]  ClampingZeroOutMax=[]  FilterDenConstantOutDataTypeStr=Inherit: Inherit via back propagation  FilterDenConstantOutMin=[]  FilterDenConstantOutMax=[]  PCopyOutDataTypeStr=Inherit: Inherit via back propagation  PCopyOutMin=[]  PCopyOutMax=[]  NCopyOutDataTypeStr=Inherit: Inherit via back propagation  NCopyOutMin=[]  NCopyOutMax=[]  IntegratorContinuousStateAttributes=''  IntegratorStateMustResolveToSignalObject=off  IntegratorRTWStateStorageClass=Auto  FilterContinuousStateAttributes=''  FilterStateMustResolveToSignalObject=off  FilterRTWStateStorageClass=Auto  ParallelPVariant=InternalParameters  IdealPVariant=Disabled  IVariant=InternalParameters  DVariant=InternalParameters  IntegratorVariant=Discrete  SatVariant=Disabled  AWVariant=Passthrough  PCopyVariant=Disabled  TRVariant=Disabled  FdbkBlocksVariant=Forward  IdealPFdbkVariant=Disabled  SatFdbkVariant=Disabled  DerivativeFilterVariant=ForwardEulerFilter  NVariant=InternalParameters  NCopyVariant=Disabled  FilterICVariant=InternalICsFilter  IntegratorICVariant=InternalICs  ExternalResetVariant=Disabled  TRSumVariant=Passthrough  SumFdbkVariant=Disabled  SumVariant=Sum_PID  TsampFilterVariant=InternalTs  TsampNgainVariant=Passthrough  TsampIntegralVariant=Disabled_SignalSpec  ExternalSaturationOutDataTypeStr=Inherit: Same as second input
  Rate Transition4 : RateTransition  OutPortSampleTime=0.01
  Rate Transition9 : RateTransition  OutPortSampleTime=0.01
  Saturation{,1,4..5} (4 alike) : Saturate  UpperLimit=3000  LowerLimit=-3000
  Saturation2 : Saturate  UpperLimit=400  LowerLimit=-400
  Saturation3 : Saturate  UpperLimit=400  LowerLimit=-400
  Saturation6 : Saturate  UpperLimit=400  LowerLimit=-400
  Scope{,1..3,5..15,18} (16 alike) : Scope
  Scope4 : Scope  NumInputPorts=2
  Subsystem : Subsystem
  Subsystem1 : Subsystem
  Subsystem2 : Subsystem
  Subsystem3 : Subsystem
  Motor1_pos_req_qc : Outport
  Force_sensor_afterOffset_1 : Outport  Port=2
  Motor2_pos_req_qc : Outport  Port=3
  Force_sensor_afterOffset_2 : Outport  Port=4
  Motor3_pos_req_qc : Outport  Port=5
  Force_sensor_afterOffset_3 : Outport  Port=6
  Motor4_pos_req_qc : Outport  Port=7
  Force_sensor_afterOffset_4 : Outport  Port=8
  wires:
  Cable_Tension_No1_mN/1 -> Manual Switch/1
  Compare To Constant3/1 -> Subsystem2/Enable
  Minus4/1 -> Scope2/1, Minus/2, Force_sensor_afterOffset_1/1
  Compare To Constant2/1 -> Subsystem/Enable
  Compare To Constant4/1 -> Subsystem3/Enable
  Subsystem3/1(Out1) -> Minus7/2, Scope7/1
  [time] -> Compare To Constant4/1
  Force_sensor_4_g/1 -> Minus7/1, Scope11/1, Subsystem3/1(encoder1)
  Force_sensor_2_g/1 -> Minus5/1, Subsystem1/1(encoder1)
  Minus2/1 -> PID Controller2/1
  Saturation6/1 -> Add2/2
  Force_sensor_3_g/1 -> Minus6/1, Subsystem2/1(encoder1), Scope10/1
  Force_sensor_1_g/1 -> Scope15/1, Minus4/1, Subsystem/1(encoder1)
  Gain/1 -> Add/1
  Gain1/1 -> Add1/1
  Add2/1 -> Saturation/1, Scope9/1
  Gain2/1 -> Add2/1
  Constant9/1 -> Manual Switch2/2
  PID Controller/1 -> Saturation6/1
  Saturation3/1 -> Add1/2
  Saturation/1 -> Motor1_pos_req_qc/1
  [time] -> Compare To Constant3/1
  PID Controller3/1 -> Saturation3/1
  Add/1 -> Saturation4/1, Scope4/1
  Cable_Tension_No2_mN/1 -> Manual Switch1/1
  Constant10/1 -> Manual Switch3/2
  Minus/1 -> PID Controller/1
  Subsystem1/1(Out1) -> Minus5/2, Scope5/1
  Analog Filter Design1/1 -> Minus1/2, Force_sensor_afterOffset_2/1
  Minus5/1 -> Analog Filter Design1/1
  Saturation1/1 -> Motor2_pos_req_qc/1
  [time] -> Compare To Constant1/1
  Cable_Tension_No3_mN/1 -> Rate Transition4/1
  Constant3/1 -> Manual Switch/2
  Saturation2/1 -> Add/2, Scope4/2
  [time] -> Compare To Constant2/1
  Manual Switch2/1 -> Minus2/1, Gain/1
  Add1/1 -> Saturation5/1
  Minus3/1 -> PID Controller3/1
  Minus7/1 -> Scope12/1, Minus3/2, Force_sensor_afterOffset_4/1
  Manual Switch/1 -> Minus/1, Gain2/1, Scope8/1
  Cable_Tension_No4_mN/1 -> Scope3/1, Manual Switch3/1
  Manual Switch1/1 -> Minus1/1
  Saturation4/1 -> Scope14/1, Motor3_pos_req_qc/1
  Minus6/1 -> Scope1/1, Minus2/2, Force_sensor_afterOffset_3/1
  PID Controller2/1 -> Saturation2/1
  Saturation5/1 -> Scope13/1, Motor4_pos_req_qc/1
  Manual Switch3/1 -> Minus3/1, Gain1/1
  PID Controller1/1 -> Saturation1/1
  Subsystem/1(Out1) -> Minus4/2, Scope/1
  Minus1/1 -> PID Controller1/1
  Compare To Constant1/1 -> Subsystem1/Enable
  Subsystem2/1(Out1) -> Minus6/2, Scope6/1
  Constant8/1 -> Manual Switch1/2
  Clock3/1 -> Rate Transition9/1
  Rate Transition9/1 -> [time]
  Rate Transition4/1 -> Minus8/1, Scope18/1
  Constant/1 -> Minus8/2
  Minus8/1 -> Manual Switch2/1
